simulink model "tuoyuan"  (R2023b)
settings: Solver=FixedStepAuto  StartTime=0.0  StopTime=15  FixedStep=1e-3  RelTol=1e-3
settings Model: Creator=asus  LastModifiedBy=asus

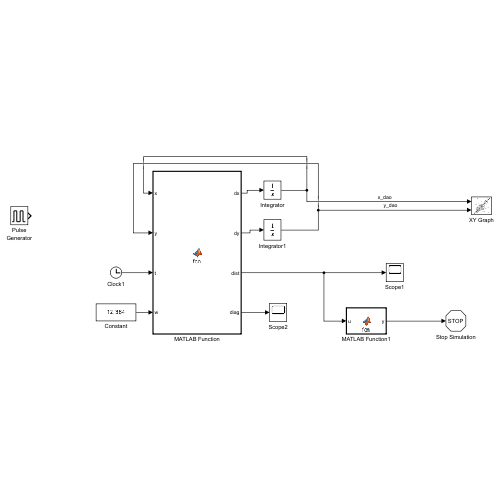
[thumbnail: Simulink's stored preview of the top-level diagram]
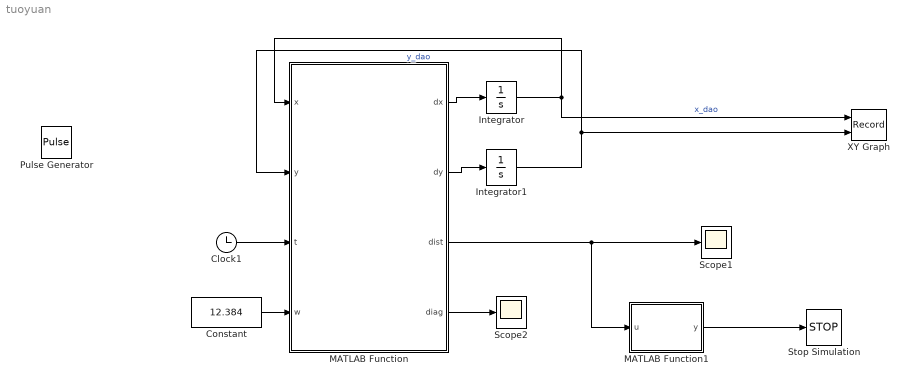
== system tuoyuan ==
  Clock1 : Clock
  Constant : Constant  Value=12.384
  Integrator : Integrator
  Integrator1 : Integrator
  MATLAB Function : MATLAB Function  TreatAsAtomicUnit=on
  MATLAB Function1 : MATLAB Function  TreatAsAtomicUnit=on
  Pulse Generator : DiscretePulseGenerator  PulseType=Time based  Period=10  PulseWidth=5
  Scope1 : Scope
  Scope2 : Scope
  Stop Simulation : Stop
  XY Graph : Record  FileSettingsInternal="{\"entries\":[{\"content\":{\"excelSettings\":{\"content\":{},\"type\":\"Streamout.ExcelSettings\"}},\"type\":\"Streamout.FileSettingStorage\",\"uuid\":\"\"}],\"packageUris\":[\"http:\\/\\/schema.mathworks.com\\/mf0\\/streamout_blocks\\/R2020a\"],\"version\":\"1.0\"}"  Layout=[1 1]  SignalsInternal="{\"entries\":[{\"content\":{\"signals\":[{\"content\":{\"blockPath\":[],\"dimensions\":[1],\"domain\":\"\",\"lineColor\":\"#a2142f\",\"plots\":[1],\"port\":1,\"sid\":[\"\"],\"signalID\":638,\"signalName\":\"x_dao\"},\"type\":\"RecordBlkView.Signal\",\"uuid\":\"\"},{\"content\":{\"blockPath\":[],\"dimensions\":[1],\"domain\":\"\",\"lineColor\":\"#139fff\",\"plots\":[1],\"port\":2,\"sid\":[\"\"],\"signalID\":642,\"signalName\":\"y_dao\"},\"type\":\"RecordBlkView.Signal\",\"uuid\":\"\"}]},\"type\":\"RecordBlkView.InputSignals\",\"uuid\":\"\"}],\"packageUris\":[\"http:\\/\\/schema.mathworks.com\\/mf0\\/streamout_blocks\\/R2020a\"],\"version\":\"1.0\"}"  VisualizationBindings="{\"xyplotplugin\":{\"info\":[{\"series\":[{\"bindingParametersList\":[{\"parameter\":\"X-Axis\",\"signalID\":638,\"signalName\":\"x_dao\"},{\"parameter\":\"Y-Axis\",\"signalID\":642,\"signalName\":\"y_dao\"}],\"seriesID\":44510}],\"subplotID\":1}]}}"  CompatibilityTag=XY
  wires:
  MATLAB Function/1(dx) -> Integrator/1
  Integrator/1 -> XY Graph/1, MATLAB Function/1(x)  "x_dao"
  Integrator1/1 -> XY Graph/2, MATLAB Function/2(y)  "y_dao"
  MATLAB Function/2(dy) -> Integrator1/1
  Clock1/1 -> MATLAB Function/3(t)
  Constant/1 -> MATLAB Function/4(w)
  MATLAB Function/4(diag) -> Scope2/1
  MATLAB Function1/1(y) -> Stop Simulation/1
  MATLAB Function/3(dist) -> MATLAB Function1/1(u), Scope1/1

== matlab function tuoyuan/MATLAB Function1 ==
  data: u input; y output
function y = fcn(u)

if(u<1e-2)
    y=1;
else
    y=0;
end

== matlab function tuoyuan/MATLAB Function ==
  data: x input; dx output; y input; t input; dy output; dist output; diag output; w input
function [dx,dy,dist,diag] = fcn(x,y,t,w)
x_fei = 10 + 20*cos(t);
y_fei = 20 + 5*sin(t);
dist = sqrt( (x_fei - x)^2 + (y_fei - y)^2 );

if(dist > 0)
    dx = w * (x_fei - x) / dist;
    dy = w * (y_fei - y) / dist;
    diag = 0;
elseif(dist == 0)
    dx=0;
    dy=0;
    diag = 1;
else
    dx=0;
    dy=0;
    diag = 2;
end
